simulink model "test4"  (R2015a)
settings: Solver=ode45  StartTime=0.0  StopTime=330000  RelTol=1e-3
InitFcn:
  | %% DSPBuilder Start
  | alt_dspbuilder_update_model(bdroot)
  | %% DSPBuilder End
libraries: allblocks_alteradspbuilder2 x840
(part 2 of 11)

== system test4/sift/Subsystem1/calculate_key_point/find_KeyPoint ==
  dataIn_10 : Inport
  dataIn_11 : Inport  Port=2
  dataIn_12 : Inport  Port=3
  dataIn_13 : Inport  Port=4
  dataIn_14 : Inport  Port=5
  dataIn_15 : Inport  Port=6
  dataIn_16 : Inport  Port=7
  dataIn_17 : Inport  Port=8
  dataIn_18 : Inport  Port=9
  dataIn_20 : Inport  Port=10
  dataIn_21 : Inport  Port=11
  dataIn_22 : Inport  Port=12
  dataIn_23 : Inport  Port=13
  dataIn_24 : Inport  Port=14
  dataIn_25 : Inport  Port=15
  dataIn_26 : Inport  Port=16
  dataIn_27 : Inport  Port=17
  dataIn_28 : Inport  Port=18
  dataIn_30 : Inport  Port=19
  dataIn_31 : Inport  Port=20
  dataIn_32 : Inport  Port=21
  dataIn_33 : Inport  Port=22
  dataIn_34 : Inport  Port=23
  dataIn_35 : Inport  Port=24
  dataIn_36 : Inport  Port=25
  dataIn_37 : Inport  Port=26
  dataIn_38 : Inport  Port=27
  Logical Bit Operator : allblocks_alteradspbuilder2/Logical Bit Operator  LogicalOperator=OR  user_inputs=2  pipeline_display=0
  find_Keymax : Subsystem
  find_min : Subsystem
  is_KeyPoint : Outport
  wires:
  [dataIn_32] -> find_Keymax/21(dataIn_32)
  [dataIn_33] -> find_Keymax/22(dataIn_33)
  [dataIn_36] -> find_Keymax/25(dataIn_36)
  [dataIn_37] -> find_Keymax/26(dataIn_37)
  [dataIn_34] -> find_Keymax/23(dataIn_34)
  [dataIn_35] -> find_Keymax/24(dataIn_35)
  [dataIn_30] -> find_Keymax/19(dataIn_30)
  [dataIn_31] -> find_Keymax/20(dataIn_31)
  [is_KeyPoint_Max] -> Logical Bit Operator/2
  [is_KeyPoint_Min] -> Logical Bit Operator/1
  find_Keymax/1(is_KeyPoint) -> [is_KeyPoint_Max]
  [dataIn_28] -> find_Keymax/18(dataIn_28)
  [dataIn_26] -> find_Keymax/16(dataIn_26)
  [dataIn_22] -> find_Keymax/12(dataIn_22)
  [dataIn_27] -> find_Keymax/17(dataIn_27)
  [dataIn_20] -> find_Keymax/10(dataIn_20)
  [dataIn_23] -> find_Keymax/13(dataIn_23)
  [dataIn_24] -> find_Keymax/14(dataIn_24)
  [dataIn_21] -> find_Keymax/11(dataIn_21)
  [dataIn_25] -> find_Keymax/15(dataIn_25)
  [dataIn_10] -> find_Keymax/1(dataIn_10)
  [dataIn_11] -> find_Keymax/2(dataIn_11)
  [dataIn_12] -> find_Keymax/3(dataIn_12)
  dataIn_23/1 -> [dataIn_23]
  dataIn_17/1 -> [dataIn_17]
  dataIn_22/1 -> [dataIn_22]
  dataIn_14/1 -> [dataIn_14]
  dataIn_16/1 -> [dataIn_16]
  dataIn_28/1 -> [dataIn_28]
  dataIn_20/1 -> [dataIn_20]
  dataIn_21/1 -> [dataIn_21]
  dataIn_26/1 -> [dataIn_26]
  dataIn_10/1 -> [dataIn_10]
  dataIn_30/1 -> [dataIn_30]
  dataIn_27/1 -> [dataIn_27]
  dataIn_25/1 -> [dataIn_25]
  dataIn_15/1 -> [dataIn_15]
  dataIn_18/1 -> [dataIn_18]
  dataIn_24/1 -> [dataIn_24]
  dataIn_32/1 -> [dataIn_32]
  dataIn_13/1 -> [dataIn_13]
  dataIn_31/1 -> [dataIn_31]
  [dataIn_14] -> find_Keymax/5(dataIn_14)
  dataIn_34/1 -> [dataIn_34]
  dataIn_11/1 -> [dataIn_11]
  [dataIn_17] -> find_Keymax/8(dataIn_17)
  dataIn_35/1 -> [dataIn_35]
  dataIn_33/1 -> [dataIn_33]
  dataIn_38/1 -> [dataIn_38]
  [dataIn_13] -> find_Keymax/4(dataIn_13)
  [dataIn_16] -> find_Keymax/7(dataIn_16)
  [dataIn_15] -> find_Keymax/6(dataIn_15)
  dataIn_12/1 -> [dataIn_12]
  [dataIn_18] -> find_Keymax/9(dataIn_18)
  dataIn_36/1 -> [dataIn_36]
  dataIn_37/1 -> [dataIn_37]
  [dataIn_38] -> find_Keymax/27(dataIn_38)
  find_min/1(is_KeyPoint) -> [is_KeyPoint_Min]
  [dataIn_11] -> find_min/2(dataIn_11)
  [dataIn_12] -> find_min/3(dataIn_12)
  [dataIn_13] -> find_min/4(dataIn_13)
  [dataIn_15] -> find_min/6(dataIn_15)
  [dataIn_16] -> find_min/7(dataIn_16)
  [dataIn_17] -> find_min/8(dataIn_17)
  [dataIn_18] -> find_min/9(dataIn_18)
  [dataIn_31] -> find_min/20(dataIn_31)
  [dataIn_14] -> find_min/5(dataIn_14)
  [is_KeyPoint] -> is_KeyPoint/1
  [dataIn_33] -> find_min/22(dataIn_33)
  [dataIn_32] -> find_min/21(dataIn_32)
  [dataIn_34] -> find_min/23(dataIn_34)
  [dataIn_35] -> find_min/24(dataIn_35)
  [dataIn_36] -> find_min/25(dataIn_36)
  [dataIn_21] -> find_min/11(dataIn_21)
  [dataIn_22] -> find_min/12(dataIn_22)
  [dataIn_23] -> find_min/13(dataIn_23)
  [dataIn_25] -> find_min/15(dataIn_25)
  [dataIn_24] -> find_min/14(dataIn_24)
  [dataIn_38] -> find_min/27(dataIn_38)
  [dataIn_20] -> find_min/10(dataIn_20)
  [dataIn_26] -> find_min/16(dataIn_26)
  [dataIn_30] -> find_min/19(dataIn_30)
  [dataIn_27] -> find_min/17(dataIn_27)
  [dataIn_37] -> find_min/26(dataIn_37)
  [dataIn_28] -> find_min/18(dataIn_28)
  [dataIn_10] -> find_min/1(dataIn_10)
  Logical Bit Operator/1 -> [is_KeyPoint]

== system test4/sift/Subsystem1/calculate_key_point/line_buff_3x3 ==
  dataIn : Inport
  clken : Inport  Port=2
  Delay : allblocks_alteradspbuilder2/Delay  pipeline=1  pipeline_display=1  ClockPhase=1  use_ena=on  use_sclr=off  allowFloatingPointOverride=on  logOutputs=off  logFile=C:\Users\ASUS\Desktop\sift_fpga_final\Octave_2\tb_test4\test4_sift_Subsystem1_calculate%5Fkey%5Fpoint_line%5Fbuff%5F3x3_Delay.fixedpointlog  use_init=off  reset_value=1
  Delay1 : allblocks_alteradspbuilder2/Delay  pipeline=1  pipeline_display=1  ClockPhase=1  use_ena=on  use_sclr=off  allowFloatingPointOverride=on  logOutputs=off  logFile=C:\Users\ASUS\Desktop\sift_fpga_final\Octave_2\tb_test4\test4_sift_Subsystem1_calculate%5Fkey%5Fpoint_line%5Fbuff%5F3x3_Delay1.fixedpointlog  use_init=off  reset_value=1
  Delay10 : allblocks_alteradspbuilder2/Delay  pipeline=1  pipeline_display=1  ClockPhase=1  use_ena=on  use_sclr=off  allowFloatingPointOverride=on  logOutputs=off  logFile=C:\Users\ASUS\Desktop\sift_fpga_final\Octave_2\tb_test4\test4_sift_Subsystem1_calculate%5Fkey%5Fpoint_line%5Fbuff%5F3x3_Delay10.fixedpointlog  use_init=off  reset_value=1
  Delay2 : allblocks_alteradspbuilder2/Delay  pipeline=1  pipeline_display=1  ClockPhase=1  use_ena=on  use_sclr=off  allowFloatingPointOverride=on  logOutputs=off  logFile=C:\Users\ASUS\Desktop\sift_fpga_final\Octave_2\tb_test4\test4_sift_Subsystem1_calculate%5Fkey%5Fpoint_line%5Fbuff%5F3x3_Delay2.fixedpointlog  use_init=off  reset_value=1
  Delay5 : allblocks_alteradspbuilder2/Delay  pipeline=1  pipeline_display=1  ClockPhase=1  use_ena=on  use_sclr=off  allowFloatingPointOverride=on  logOutputs=off  logFile=C:\Users\ASUS\Desktop\sift_fpga_final\Octave_2\tb_test4\test4_sift_Subsystem1_calculate%5Fkey%5Fpoint_line%5Fbuff%5F3x3_Delay5.fixedpointlog  use_init=off  reset_value=1
  Delay6 : allblocks_alteradspbuilder2/Delay  pipeline=1  pipeline_display=1  ClockPhase=1  use_ena=on  use_sclr=off  allowFloatingPointOverride=on  logOutputs=off  logFile=C:\Users\ASUS\Desktop\sift_fpga_final\Octave_2\tb_test4\test4_sift_Subsystem1_calculate%5Fkey%5Fpoint_line%5Fbuff%5F3x3_Delay6.fixedpointlog  use_init=off  reset_value=1
  Delay9 : allblocks_alteradspbuilder2/Delay  pipeline=1  pipeline_display=1  ClockPhase=1  use_ena=on  use_sclr=off  allowFloatingPointOverride=on  logOutputs=off  logFile=C:\Users\ASUS\Desktop\sift_fpga_final\Octave_2\tb_test4\test4_sift_Subsystem1_calculate%5Fkey%5Fpoint_line%5Fbuff%5F3x3_Delay9.fixedpointlog  use_init=off  reset_value=1
  Memory Delay : allblocks_alteradspbuilder2/Memory Delay  BusType=Signed Integer  bwl=9  bwr=16  pipeline=318  pipeline_display=318  ram_type=AUTO  use_ena=on  use_sclr=off  allowFloatingPointOverride=on  logOutputs=off  logFile=C:\Users\ASUS\Desktop\sift_fpga_final\Octave_2\tb_test4\test4_sift_Subsystem1_calculate%5Fkey%5Fpoint_line%5Fbuff%5F3x3_Memory+Delay.fixedpointlog
  Memory Delay1 : allblocks_alteradspbuilder2/Memory Delay  BusType=Signed Integer  bwl=9  bwr=16  pipeline=318  pipeline_display=318  ram_type=AUTO  use_ena=on  use_sclr=off  allowFloatingPointOverride=on  logOutputs=off  logFile=C:\Users\ASUS\Desktop\sift_fpga_final\Octave_2\tb_test4\test4_sift_Subsystem1_calculate%5Fkey%5Fpoint_line%5Fbuff%5F3x3_Memory+Delay1.fixedpointlog
  Out00 : Outport
  Out01 : Outport  Port=2
  Out02 : Outport  Port=3
  Out10 : Outport  Port=4
  Out11 : Outport  Port=5
  Out12 : Outport  Port=6
  Out20 : Outport  Port=7
  Out21 : Outport  Port=8
  Out22 : Outport  Port=9
  wires:
  Delay1/1 -> [data_01], Delay2/1
  Delay/1 -> [data_00], Delay1/1
  Delay9/1 -> [data_21], Delay10/1
  [clken] -> Delay10/2
  [clken] -> Memory Delay1/2
  Delay6/1 -> Memory Delay1/1, [data_12]
  Memory Delay1/1 -> [data_20], Delay9/1
  [clken] -> Delay9/2
  [data_02] -> Out02/1
  [clken] -> Delay1/2
  [clken] -> Delay/2
  [data_in] -> Delay/1
  [clken] -> Delay2/2
  Delay2/1 -> Memory Delay/1, [data_02]
  [data_22] -> Out22/1
  Delay10/1 -> [data_22]
  clken/1 -> [clken]
  [data_21] -> Out21/1
  [data_20] -> Out20/1
  [data_10] -> Out10/1
  Memory Delay/1 -> [data_10], Delay5/1
  [clken] -> Memory Delay/2
  [clken] -> Delay6/2
  Delay5/1 -> [data_11], Delay6/1
  [data_12] -> Out12/1
  [data_00] -> Out00/1
  [data_01] -> Out01/1
  [clken] -> Delay5/2
  [data_11] -> Out11/1
  dataIn/1 -> [data_in]

== system test4/sift/Subsystem1/calculate_key_point/line_buff_3x3(1) ==
  dataIn : Inport
  clken : Inport  Port=2
  Delay : allblocks_alteradspbuilder2/Delay  pipeline=1  pipeline_display=1  ClockPhase=1  use_ena=on  use_sclr=off  allowFloatingPointOverride=on  logOutputs=off  logFile=C:\Users\ASUS\Desktop\sift_fpga_final\Octave_2\tb_test4\test4_sift_Subsystem1_calculate%5Fkey%5Fpoint_line%5Fbuff%5F3x3%281%29_Delay.fixedpointlog  use_init=off  reset_value=1
  Delay1 : allblocks_alteradspbuilder2/Delay  pipeline=1  pipeline_display=1  ClockPhase=1  use_ena=on  use_sclr=off  allowFloatingPointOverride=on  logOutputs=off  logFile=C:\Users\ASUS\Desktop\sift_fpga_final\Octave_2\tb_test4\test4_sift_Subsystem1_calculate%5Fkey%5Fpoint_line%5Fbuff%5F3x3%281%29_Delay1.fixedpointlog  use_init=off  reset_value=1
  Delay10 : allblocks_alteradspbuilder2/Delay  pipeline=1  pipeline_display=1  ClockPhase=1  use_ena=on  use_sclr=off  allowFloatingPointOverride=on  logOutputs=off  logFile=C:\Users\ASUS\Desktop\sift_fpga_final\Octave_2\tb_test4\test4_sift_Subsystem1_calculate%5Fkey%5Fpoint_line%5Fbuff%5F3x3%281%29_Delay10.fixedpointlog  use_init=off  reset_value=1
  Delay2 : allblocks_alteradspbuilder2/Delay  pipeline=1  pipeline_display=1  ClockPhase=1  use_ena=on  use_sclr=off  allowFloatingPointOverride=on  logOutputs=off  logFile=C:\Users\ASUS\Desktop\sift_fpga_final\Octave_2\tb_test4\test4_sift_Subsystem1_calculate%5Fkey%5Fpoint_line%5Fbuff%5F3x3%281%29_Delay2.fixedpointlog  use_init=off  reset_value=1
  Delay5 : allblocks_alteradspbuilder2/Delay  pipeline=1  pipeline_display=1  ClockPhase=1  use_ena=on  use_sclr=off  allowFloatingPointOverride=on  logOutputs=off  logFile=C:\Users\ASUS\Desktop\sift_fpga_final\Octave_2\tb_test4\test4_sift_Subsystem1_calculate%5Fkey%5Fpoint_line%5Fbuff%5F3x3%281%29_Delay5.fixedpointlog  use_init=off  reset_value=1
  Delay6 : allblocks_alteradspbuilder2/Delay  pipeline=1  pipeline_display=1  ClockPhase=1  use_ena=on  use_sclr=off  allowFloatingPointOverride=on  logOutputs=off  logFile=C:\Users\ASUS\Desktop\sift_fpga_final\Octave_2\tb_test4\test4_sift_Subsystem1_calculate%5Fkey%5Fpoint_line%5Fbuff%5F3x3%281%29_Delay6.fixedpointlog  use_init=off  reset_value=1
  Delay9 : allblocks_alteradspbuilder2/Delay  pipeline=1  pipeline_display=1  ClockPhase=1  use_ena=on  use_sclr=off  allowFloatingPointOverride=on  logOutputs=off  logFile=C:\Users\ASUS\Desktop\sift_fpga_final\Octave_2\tb_test4\test4_sift_Subsystem1_calculate%5Fkey%5Fpoint_line%5Fbuff%5F3x3%281%29_Delay9.fixedpointlog  use_init=off  reset_value=1
  Memory Delay : allblocks_alteradspbuilder2/Memory Delay  BusType=Signed Integer  bwl=9  bwr=16  pipeline=318  pipeline_display=318  ram_type=AUTO  use_ena=on  use_sclr=off  allowFloatingPointOverride=on  logOutputs=off  logFile=C:\Users\ASUS\Desktop\sift_fpga_final\Octave_2\tb_test4\test4_sift_Subsystem1_calculate%5Fkey%5Fpoint_line%5Fbuff%5F3x3%281%29_Memory+Delay.fixedpointlog
  Memory Delay1 : allblocks_alteradspbuilder2/Memory Delay  BusType=Signed Integer  bwl=9  bwr=16  pipeline=318  pipeline_display=318  ram_type=AUTO  use_ena=on  use_sclr=off  allowFloatingPointOverride=on  logOutputs=off  logFile=C:\Users\ASUS\Desktop\sift_fpga_final\Octave_2\tb_test4\test4_sift_Subsystem1_calculate%5Fkey%5Fpoint_line%5Fbuff%5F3x3%281%29_Memory+Delay1.fixedpointlog
  Out00 : Outport
  Out01 : Outport  Port=2
  Out02 : Outport  Port=3
  Out10 : Outport  Port=4
  Out11 : Outport  Port=5
  Out12 : Outport  Port=6
  Out20 : Outport  Port=7
  Out21 : Outport  Port=8
  Out22 : Outport  Port=9
  wires:
  Delay1/1 -> [data_01], Delay2/1
  Delay/1 -> [data_00], Delay1/1
  Delay9/1 -> [data_21], Delay10/1
  [clken] -> Delay10/2
  [clken] -> Memory Delay1/2
  Delay6/1 -> Memory Delay1/1, [data_12]
  Memory Delay1/1 -> [data_20], Delay9/1
  [clken] -> Delay9/2
  [data_02] -> Out02/1
  [clken] -> Delay1/2
  [clken] -> Delay/2
  [data_in] -> Delay/1
  [clken] -> Delay2/2
  Delay2/1 -> Memory Delay/1, [data_02]
  [data_22] -> Out22/1
  Delay10/1 -> [data_22]
  clken/1 -> [clken]
  [data_21] -> Out21/1
  [data_20] -> Out20/1
  [data_10] -> Out10/1
  Memory Delay/1 -> [data_10], Delay5/1
  [clken] -> Memory Delay/2
  [clken] -> Delay6/2
  Delay5/1 -> [data_11], Delay6/1
  [data_12] -> Out12/1
  [data_00] -> Out00/1
  [data_01] -> Out01/1
  [clken] -> Delay5/2
  [data_11] -> Out11/1
  dataIn/1 -> [data_in]

== system test4/sift/Subsystem1/calculate_key_point/line_buff_3x3(2) ==
  dataIn : Inport
  clken : Inport  Port=2
  Delay : allblocks_alteradspbuilder2/Delay  pipeline=1  pipeline_display=1  ClockPhase=1  use_ena=on  use_sclr=off  allowFloatingPointOverride=on  logOutputs=off  logFile=C:\Users\ASUS\Desktop\sift_fpga_final\Octave_2\tb_test4\test4_sift_Subsystem1_calculate%5Fkey%5Fpoint_line%5Fbuff%5F3x3%282%29_Delay.fixedpointlog  use_init=off  reset_value=1
  Delay1 : allblocks_alteradspbuilder2/Delay  pipeline=1  pipeline_display=1  ClockPhase=1  use_ena=on  use_sclr=off  allowFloatingPointOverride=on  logOutputs=off  logFile=C:\Users\ASUS\Desktop\sift_fpga_final\Octave_2\tb_test4\test4_sift_Subsystem1_calculate%5Fkey%5Fpoint_line%5Fbuff%5F3x3%282%29_Delay1.fixedpointlog  use_init=off  reset_value=1
  Delay10 : allblocks_alteradspbuilder2/Delay  pipeline=1  pipeline_display=1  ClockPhase=1  use_ena=on  use_sclr=off  allowFloatingPointOverride=on  logOutputs=off  logFile=C:\Users\ASUS\Desktop\sift_fpga_final\Octave_2\tb_test4\test4_sift_Subsystem1_calculate%5Fkey%5Fpoint_line%5Fbuff%5F3x3%282%29_Delay10.fixedpointlog  use_init=off  reset_value=1
  Delay2 : allblocks_alteradspbuilder2/Delay  pipeline=1  pipeline_display=1  ClockPhase=1  use_ena=on  use_sclr=off  allowFloatingPointOverride=on  logOutputs=off  logFile=C:\Users\ASUS\Desktop\sift_fpga_final\Octave_2\tb_test4\test4_sift_Subsystem1_calculate%5Fkey%5Fpoint_line%5Fbuff%5F3x3%282%29_Delay2.fixedpointlog  use_init=off  reset_value=1
  Delay5 : allblocks_alteradspbuilder2/Delay  pipeline=1  pipeline_display=1  ClockPhase=1  use_ena=on  use_sclr=off  allowFloatingPointOverride=on  logOutputs=off  logFile=C:\Users\ASUS\Desktop\sift_fpga_final\Octave_2\tb_test4\test4_sift_Subsystem1_calculate%5Fkey%5Fpoint_line%5Fbuff%5F3x3%282%29_Delay5.fixedpointlog  use_init=off  reset_value=1
  Delay6 : allblocks_alteradspbuilder2/Delay  pipeline=1  pipeline_display=1  ClockPhase=1  use_ena=on  use_sclr=off  allowFloatingPointOverride=on  logOutputs=off  logFile=C:\Users\ASUS\Desktop\sift_fpga_final\Octave_2\tb_test4\test4_sift_Subsystem1_calculate%5Fkey%5Fpoint_line%5Fbuff%5F3x3%282%29_Delay6.fixedpointlog  use_init=off  reset_value=1
  Delay9 : allblocks_alteradspbuilder2/Delay  pipeline=1  pipeline_display=1  ClockPhase=1  use_ena=on  use_sclr=off  allowFloatingPointOverride=on  logOutputs=off  logFile=C:\Users\ASUS\Desktop\sift_fpga_final\Octave_2\tb_test4\test4_sift_Subsystem1_calculate%5Fkey%5Fpoint_line%5Fbuff%5F3x3%282%29_Delay9.fixedpointlog  use_init=off  reset_value=1
  Memory Delay : allblocks_alteradspbuilder2/Memory Delay  BusType=Signed Integer  bwl=9  bwr=16  pipeline=318  pipeline_display=318  ram_type=AUTO  use_ena=on  use_sclr=off  allowFloatingPointOverride=on  logOutputs=off  logFile=C:\Users\ASUS\Desktop\sift_fpga_final\Octave_2\tb_test4\test4_sift_Subsystem1_calculate%5Fkey%5Fpoint_line%5Fbuff%5F3x3%282%29_Memory+Delay.fixedpointlog
  Memory Delay1 : allblocks_alteradspbuilder2/Memory Delay  BusType=Signed Integer  bwl=9  bwr=16  pipeline=318  pipeline_display=318  ram_type=AUTO  use_ena=on  use_sclr=off  allowFloatingPointOverride=on  logOutputs=off  logFile=C:\Users\ASUS\Desktop\sift_fpga_final\Octave_2\tb_test4\test4_sift_Subsystem1_calculate%5Fkey%5Fpoint_line%5Fbuff%5F3x3%282%29_Memory+Delay1.fixedpointlog
  Out00 : Outport
  Out01 : Outport  Port=2
  Out02 : Outport  Port=3
  Out10 : Outport  Port=4
  Out11 : Outport  Port=5
  Out12 : Outport  Port=6
  Out20 : Outport  Port=7
  Out21 : Outport  Port=8
  Out22 : Outport  Port=9
  wires:
  Delay1/1 -> [data_01], Delay2/1
  Delay/1 -> [data_00], Delay1/1
  Delay9/1 -> [data_21], Delay10/1
  [clken] -> Delay10/2
  [clken] -> Memory Delay1/2
  Delay6/1 -> Memory Delay1/1, [data_12]
  Memory Delay1/1 -> [data_20], Delay9/1
  [clken] -> Delay9/2
  [data_02] -> Out02/1
  [clken] -> Delay1/2
  [clken] -> Delay/2
  [data_in] -> Delay/1
  [clken] -> Delay2/2
  Delay2/1 -> Memory Delay/1, [data_02]
  [data_22] -> Out22/1
  Delay10/1 -> [data_22]
  clken/1 -> [clken]
  [data_21] -> Out21/1
  [data_20] -> Out20/1
  [data_10] -> Out10/1
  Memory Delay/1 -> [data_10], Delay5/1
  [clken] -> Memory Delay/2
  [clken] -> Delay6/2
  Delay5/1 -> [data_11], Delay6/1
  [data_12] -> Out12/1
  [data_00] -> Out00/1
  [data_01] -> Out01/1
  [clken] -> Delay5/2
  [data_11] -> Out11/1
  dataIn/1 -> [data_in]

== system test4/sift/Subsystem1/scale_space/Gaussian_scale1 ==
  pixel_in : Inport
  valid_in : Inport  Port=2
  Mul : Subsystem
  Round : allblocks_alteradspbuilder2/Round  BusType=Signed Fractional  bwl=9  bwr=16  bitsToRemove=0  roundMode=TRUNCATE_LOW  userRoundMode=Truncate  pipeline=off  pipeline_display=0  use_ena=off  use_aclr=off
  line_buff : Subsystem
  pixel_out : Outport
  wires:
  line_buff/20(Out34) -> Mul/20(In34)
  line_buff/7(Out11) -> Mul/7(In11)
  line_buff/22(Out41) -> Mul/22(In41)
  line_buff/21(Out40) -> Mul/21(In40)
  line_buff/23(Out42) -> Mul/23(In42)
  line_buff/24(Out43) -> Mul/24(In43)
  line_buff/6(Out10) -> Mul/6(In10)
  line_buff/19(Out33) -> Mul/19(In33)
  line_buff/25(Out44) -> Mul/25(In44)
  line_buff/11(Out20) -> Mul/11(In20)
  line_buff/1(Out00) -> Mul/1(In00)
  line_buff/5(Out04) -> Mul/5(In04)
  pixel_in/1 -> line_buff/1(dataIn)
  line_buff/13(Out22) -> Mul/13(In22)
  line_buff/16(Out30) -> Mul/16(In30)
  line_buff/18(Out32) -> Mul/18(In32)
  Mul/1(pixel) -> Round/1
  line_buff/10(Out14) -> Mul/10(In14)
  valid_in/1 -> Mul/26(clken), line_buff/2(clken)
  line_buff/12(Out21) -> Mul/12(In21)
  line_buff/14(Out23) -> Mul/14(In23)
  line_buff/2(Out01) -> Mul/2(In01)
  line_buff/4(Out03) -> Mul/4(In03)
  line_buff/9(Out13) -> Mul/9(In13)
  line_buff/15(Out24) -> Mul/15(In24)
  line_buff/17(Out31) -> Mul/17(In31)
  line_buff/3(Out02) -> Mul/3(In02)
  line_buff/8(Out12) -> Mul/8(In12)
  Round/1 -> pixel_out/1

== system test4/sift/Subsystem1/scale_space/Gaussian_scale2 ==
  pixel_in : Inport
  valid_in : Inport  Port=2
  Mul : Subsystem
  Round : allblocks_alteradspbuilder2/Round  BusType=Signed Fractional  bwl=9  bwr=16  bitsToRemove=0  roundMode=TRUNCATE_LOW  userRoundMode=Truncate  pipeline=off  pipeline_display=0  use_ena=off  use_aclr=off
  line_buff : Subsystem
  pixel_out : Outport
  wires:
  line_buff/20(Out34) -> Mul/20(In34)
  line_buff/7(Out11) -> Mul/7(In11)
  line_buff/22(Out41) -> Mul/22(In41)
  line_buff/21(Out40) -> Mul/21(In40)
  line_buff/23(Out42) -> Mul/23(In42)
  line_buff/24(Out43) -> Mul/24(In43)
  line_buff/6(Out10) -> Mul/6(In10)
  line_buff/19(Out33) -> Mul/19(In33)
  line_buff/25(Out44) -> Mul/25(In44)
  line_buff/11(Out20) -> Mul/11(In20)
  line_buff/1(Out00) -> Mul/1(In00)
  line_buff/5(Out04) -> Mul/5(In04)
  pixel_in/1 -> line_buff/1(dataIn)
  line_buff/13(Out22) -> Mul/13(In22)
  line_buff/16(Out30) -> Mul/16(In30)
  line_buff/18(Out32) -> Mul/18(In32)
  Mul/1(pixel) -> Round/1
  line_buff/10(Out14) -> Mul/10(In14)
  valid_in/1 -> Mul/26(clken), line_buff/2(clken)
  line_buff/12(Out21) -> Mul/12(In21)
  line_buff/14(Out23) -> Mul/14(In23)
  line_buff/2(Out01) -> Mul/2(In01)
  line_buff/4(Out03) -> Mul/4(In03)
  line_buff/9(Out13) -> Mul/9(In13)
  line_buff/15(Out24) -> Mul/15(In24)
  line_buff/17(Out31) -> Mul/17(In31)
  line_buff/3(Out02) -> Mul/3(In02)
  line_buff/8(Out12) -> Mul/8(In12)
  Round/1 -> pixel_out/1

== system test4/sift/Subsystem1/scale_space/Gaussian_scale3 ==
  pixel_in : Inport
  valid_in : Inport  Port=2
  Mul : Subsystem
  Round : allblocks_alteradspbuilder2/Round  BusType=Signed Fractional  bwl=9  bwr=16  bitsToRemove=0  roundMode=TRUNCATE_LOW  userRoundMode=Truncate  pipeline=off  pipeline_display=0  use_ena=off  use_aclr=off
  line_buff : Subsystem
  pixel_out : Outport
  wires:
  line_buff/20(Out34) -> Mul/20(In34)
  line_buff/7(Out11) -> Mul/7(In11)
  line_buff/22(Out41) -> Mul/22(In41)
  line_buff/21(Out40) -> Mul/21(In40)
  line_buff/23(Out42) -> Mul/23(In42)
  line_buff/24(Out43) -> Mul/24(In43)
  line_buff/6(Out10) -> Mul/6(In10)
  line_buff/19(Out33) -> Mul/19(In33)
  line_buff/25(Out44) -> Mul/25(In44)
  line_buff/11(Out20) -> Mul/11(In20)
  line_buff/1(Out00) -> Mul/1(In00)
  line_buff/5(Out04) -> Mul/5(In04)
  pixel_in/1 -> line_buff/1(dataIn)
  line_buff/13(Out22) -> Mul/13(In22)
  line_buff/16(Out30) -> Mul/16(In30)
  line_buff/18(Out32) -> Mul/18(In32)
  Mul/1(pixel) -> Round/1
  line_buff/10(Out14) -> Mul/10(In14)
  valid_in/1 -> Mul/26(clken), line_buff/2(clken)
  line_buff/12(Out21) -> Mul/12(In21)
  line_buff/14(Out23) -> Mul/14(In23)
  line_buff/2(Out01) -> Mul/2(In01)
  line_buff/4(Out03) -> Mul/4(In03)
  line_buff/9(Out13) -> Mul/9(In13)
  line_buff/15(Out24) -> Mul/15(In24)
  line_buff/17(Out31) -> Mul/17(In31)
  line_buff/3(Out02) -> Mul/3(In02)
  line_buff/8(Out12) -> Mul/8(In12)
  Round/1 -> pixel_out/1

== system test4/sift/Subsystem1/scale_space/Gaussian_scale4 ==
  pixel_in : Inport
  valid_in : Inport  Port=2
  Mul : Subsystem
  Round : allblocks_alteradspbuilder2/Round  BusType=Signed Fractional  bwl=9  bwr=16  bitsToRemove=0  roundMode=TRUNCATE_LOW  userRoundMode=Truncate  pipeline=off  pipeline_display=0  use_ena=off  use_aclr=off
  line_buff : Subsystem
  pixel_out : Outport
  wires:
  line_buff/20(Out34) -> Mul/20(In34)
  line_buff/7(Out11) -> Mul/7(In11)
  line_buff/22(Out41) -> Mul/22(In41)
  line_buff/21(Out40) -> Mul/21(In40)
  line_buff/23(Out42) -> Mul/23(In42)
  line_buff/24(Out43) -> Mul/24(In43)
  line_buff/6(Out10) -> Mul/6(In10)
  line_buff/19(Out33) -> Mul/19(In33)
  line_buff/25(Out44) -> Mul/25(In44)
  line_buff/11(Out20) -> Mul/11(In20)
  line_buff/1(Out00) -> Mul/1(In00)
  line_buff/5(Out04) -> Mul/5(In04)
  pixel_in/1 -> line_buff/1(dataIn)
  line_buff/13(Out22) -> Mul/13(In22)
  line_buff/16(Out30) -> Mul/16(In30)
  line_buff/18(Out32) -> Mul/18(In32)
  Mul/1(pixel) -> Round/1
  line_buff/10(Out14) -> Mul/10(In14)
  valid_in/1 -> Mul/26(clken), line_buff/2(clken)
  line_buff/12(Out21) -> Mul/12(In21)
  line_buff/14(Out23) -> Mul/14(In23)
  line_buff/2(Out01) -> Mul/2(In01)
  line_buff/4(Out03) -> Mul/4(In03)
  line_buff/9(Out13) -> Mul/9(In13)
  line_buff/15(Out24) -> Mul/15(In24)
  line_buff/17(Out31) -> Mul/17(In31)
  line_buff/3(Out02) -> Mul/3(In02)
  line_buff/8(Out12) -> Mul/8(In12)
  Round/1 -> pixel_out/1

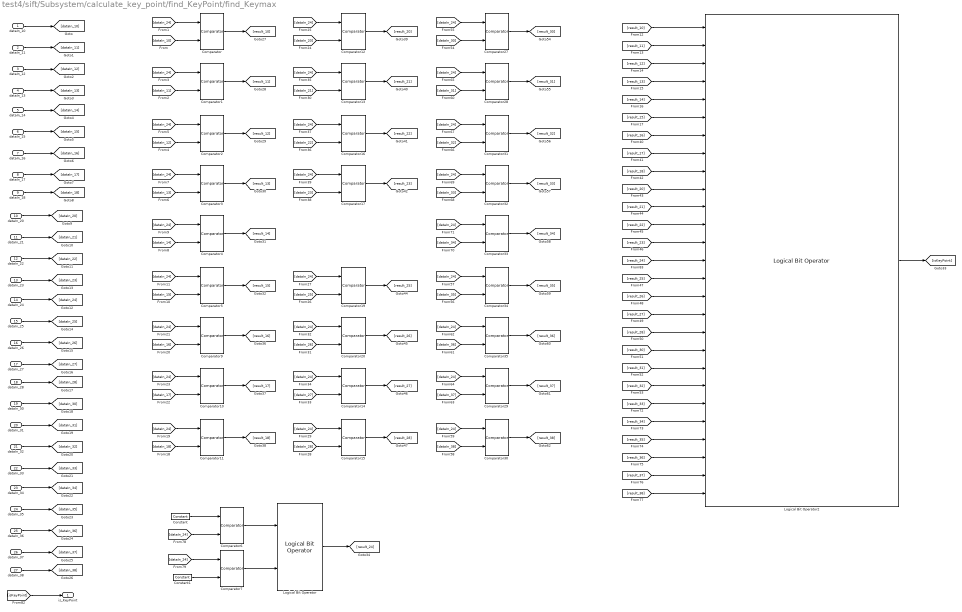
== system test4/sift/Subsystem/calculate_key_point/find_KeyPoint/find_Keymax ==
  dataIn_10 : Inport
  dataIn_11 : Inport  Port=2
  dataIn_12 : Inport  Port=3
  dataIn_13 : Inport  Port=4
  dataIn_14 : Inport  Port=5
  dataIn_15 : Inport  Port=6
  dataIn_16 : Inport  Port=7
  dataIn_17 : Inport  Port=8
  dataIn_18 : Inport  Port=9
  dataIn_20 : Inport  Port=10
  dataIn_21 : Inport  Port=11
  dataIn_22 : Inport  Port=12
  dataIn_23 : Inport  Port=13
  dataIn_24 : Inport  Port=14
  dataIn_25 : Inport  Port=15
  dataIn_26 : Inport  Port=16
  dataIn_27 : Inport  Port=17
  dataIn_28 : Inport  Port=18
  dataIn_30 : Inport  Port=19
  dataIn_31 : Inport  Port=20
  dataIn_32 : Inport  Port=21
  dataIn_33 : Inport  Port=22
  dataIn_34 : Inport  Port=23
  dataIn_35 : Inport  Port=24
  dataIn_36 : Inport  Port=25
  dataIn_37 : Inport  Port=26
  dataIn_38 : Inport  Port=27
  Comparator : allblocks_alteradspbuilder2/Comparator  direction=a > b  pipeline_display=0  allowFloatingPointOverride=on  logOutputs=off  logFile=C:\Users\ASUS\Desktop\sift_fpga_final\Octave_2\tb_test4\test4_sift_Subsystem_calculate%5Fkey%5Fpoint_find%5FKeyPoint_find%5FKeymax_Comparator.fixedpointlog
  Comparator1 : allblocks_alteradspbuilder2/Comparator  direction=a > b  pipeline_display=0  allowFloatingPointOverride=on  logOutputs=off  logFile=C:\Users\ASUS\Desktop\sift_fpga_final\Octave_2\tb_test4\test4_sift_Subsystem_calculate%5Fkey%5Fpoint_find%5FKeyPoint_find%5FKeymax_Comparator1.fixedpointlog
  Comparator10 : allblocks_alteradspbuilder2/Comparator  direction=a > b  pipeline_display=0  allowFloatingPointOverride=on  logOutputs=off  logFile=C:\Users\ASUS\Desktop\sift_fpga_final\Octave_2\tb_test4\test4_sift_Subsystem_calculate%5Fkey%5Fpoint_find%5FKeyPoint_find%5FKeymax_Comparator10.fixedpointlog
  Comparator11 : allblocks_alteradspbuilder2/Comparator  direction=a > b  pipeline_display=0  allowFloatingPointOverride=on  logOutputs=off  logFile=C:\Users\ASUS\Desktop\sift_fpga_final\Octave_2\tb_test4\test4_sift_Subsystem_calculate%5Fkey%5Fpoint_find%5FKeyPoint_find%5FKeymax_Comparator11.fixedpointlog
  Comparator12 : allblocks_alteradspbuilder2/Comparator  direction=a > b  pipeline_display=0  allowFloatingPointOverride=on  logOutputs=off  logFile=C:\Users\ASUS\Desktop\sift_fpga_final\Octave_2\tb_test4\test4_sift_Subsystem_calculate%5Fkey%5Fpoint_find%5FKeyPoint_find%5FKeymax_Comparator12.fixedpointlog
  Comparator13 : allblocks_alteradspbuilder2/Comparator  direction=a > b  pipeline_display=0  allowFloatingPointOverride=on  logOutputs=off  logFile=C:\Users\ASUS\Desktop\sift_fpga_final\Octave_2\tb_test4\test4_sift_Subsystem_calculate%5Fkey%5Fpoint_find%5FKeyPoint_find%5FKeymax_Comparator13.fixedpointlog
  Comparator14 : allblocks_alteradspbuilder2/Comparator  direction=a > b  pipeline_display=0  allowFloatingPointOverride=on  logOutputs=off  logFile=C:\Users\ASUS\Desktop\sift_fpga_final\Octave_2\tb_test4\test4_sift_Subsystem_calculate%5Fkey%5Fpoint_find%5FKeyPoint_find%5FKeymax_Comparator14.fixedpointlog
  Comparator15 : allblocks_alteradspbuilder2/Comparator  direction=a > b  pipeline_display=0  allowFloatingPointOverride=on  logOutputs=off  logFile=C:\Users\ASUS\Desktop\sift_fpga_final\Octave_2\tb_test4\test4_sift_Subsystem_calculate%5Fkey%5Fpoint_find%5FKeyPoint_find%5FKeymax_Comparator15.fixedpointlog
  Comparator16 : allblocks_alteradspbuilder2/Comparator  direction=a > b  pipeline_display=0  allowFloatingPointOverride=on  logOutputs=off  logFile=C:\Users\ASUS\Desktop\sift_fpga_final\Octave_2\tb_test4\test4_sift_Subsystem_calculate%5Fkey%5Fpoint_find%5FKeyPoint_find%5FKeymax_Comparator16.fixedpointlog
  Comparator17 : allblocks_alteradspbuilder2/Comparator  direction=a > b  pipeline_display=0  allowFloatingPointOverride=on  logOutputs=off  logFile=C:\Users\ASUS\Desktop\sift_fpga_final\Octave_2\tb_test4\test4_sift_Subsystem_calculate%5Fkey%5Fpoint_find%5FKeyPoint_find%5FKeymax_Comparator17.fixedpointlog
  Comparator19 : allblocks_alteradspbuilder2/Comparator  direction=a > b  pipeline_display=0  allowFloatingPointOverride=on  logOutputs=off  logFile=C:\Users\ASUS\Desktop\sift_fpga_final\Octave_2\tb_test4\test4_sift_Subsystem_calculate%5Fkey%5Fpoint_find%5FKeyPoint_find%5FKeymax_Comparator19.fixedpointlog
  Comparator2 : allblocks_alteradspbuilder2/Comparator  direction=a > b  pipeline_display=0  allowFloatingPointOverride=on  logOutputs=off  logFile=C:\Users\ASUS\Desktop\sift_fpga_final\Octave_2\tb_test4\test4_sift_Subsystem_calculate%5Fkey%5Fpoint_find%5FKeyPoint_find%5FKeymax_Comparator2.fixedpointlog
  Comparator20 : allblocks_alteradspbuilder2/Comparator  direction=a > b  pipeline_display=0  allowFloatingPointOverride=on  logOutputs=off  logFile=C:\Users\ASUS\Desktop\sift_fpga_final\Octave_2\tb_test4\test4_sift_Subsystem_calculate%5Fkey%5Fpoint_find%5FKeyPoint_find%5FKeymax_Comparator20.fixedpointlog
  Comparator27 : allblocks_alteradspbuilder2/Comparator  direction=a > b  pipeline_display=0  allowFloatingPointOverride=on  logOutputs=off  logFile=C:\Users\ASUS\Desktop\sift_fpga_final\Octave_2\tb_test4\test4_sift_Subsystem_calculate%5Fkey%5Fpoint_find%5FKeyPoint_find%5FKeymax_Comparator27.fixedpointlog
  Comparator28 : allblocks_alteradspbuilder2/Comparator  direction=a > b  pipeline_display=0  allowFloatingPointOverride=on  logOutputs=off  logFile=C:\Users\ASUS\Desktop\sift_fpga_final\Octave_2\tb_test4\test4_sift_Subsystem_calculate%5Fkey%5Fpoint_find%5FKeyPoint_find%5FKeymax_Comparator28.fixedpointlog
  Comparator29 : allblocks_alteradspbuilder2/Comparator  direction=a > b  pipeline_display=0  allowFloatingPointOverride=on  logOutputs=off  logFile=C:\Users\ASUS\Desktop\sift_fpga_final\Octave_2\tb_test4\test4_sift_Subsystem_calculate%5Fkey%5Fpoint_find%5FKeyPoint_find%5FKeymax_Comparator29.fixedpointlog
  Comparator3 : allblocks_alteradspbuilder2/Comparator  direction=a > b  pipeline_display=0  allowFloatingPointOverride=on  logOutputs=off  logFile=C:\Users\ASUS\Desktop\sift_fpga_final\Octave_2\tb_test4\test4_sift_Subsystem_calculate%5Fkey%5Fpoint_find%5FKeyPoint_find%5FKeymax_Comparator3.fixedpointlog
  Comparator30 : allblocks_alteradspbuilder2/Comparator  direction=a > b  pipeline_display=0  allowFloatingPointOverride=on  logOutputs=off  logFile=C:\Users\ASUS\Desktop\sift_fpga_final\Octave_2\tb_test4\test4_sift_Subsystem_calculate%5Fkey%5Fpoint_find%5FKeyPoint_find%5FKeymax_Comparator30.fixedpointlog
  Comparator31 : allblocks_alteradspbuilder2/Comparator  direction=a > b  pipeline_display=0  allowFloatingPointOverride=on  logOutputs=off  logFile=C:\Users\ASUS\Desktop\sift_fpga_final\Octave_2\tb_test4\test4_sift_Subsystem_calculate%5Fkey%5Fpoint_find%5FKeyPoint_find%5FKeymax_Comparator31.fixedpointlog
  Comparator32 : allblocks_alteradspbuilder2/Comparator  direction=a > b  pipeline_display=0  allowFloatingPointOverride=on  logOutputs=off  logFile=C:\Users\ASUS\Desktop\sift_fpga_final\Octave_2\tb_test4\test4_sift_Subsystem_calculate%5Fkey%5Fpoint_find%5FKeyPoint_find%5FKeymax_Comparator32.fixedpointlog
  Comparator33 : allblocks_alteradspbuilder2/Comparator  direction=a > b  pipeline_display=0  allowFloatingPointOverride=on  logOutputs=off  logFile=C:\Users\ASUS\Desktop\sift_fpga_final\Octave_2\tb_test4\test4_sift_Subsystem_calculate%5Fkey%5Fpoint_find%5FKeyPoint_find%5FKeymax_Comparator33.fixedpointlog
  Comparator34 : allblocks_alteradspbuilder2/Comparator  direction=a > b  pipeline_display=0  allowFloatingPointOverride=on  logOutputs=off  logFile=C:\Users\ASUS\Desktop\sift_fpga_final\Octave_2\tb_test4\test4_sift_Subsystem_calculate%5Fkey%5Fpoint_find%5FKeyPoint_find%5FKeymax_Comparator34.fixedpointlog
  Comparator35 : allblocks_alteradspbuilder2/Comparator  direction=a > b  pipeline_display=0  allowFloatingPointOverride=on  logOutputs=off  logFile=C:\Users\ASUS\Desktop\sift_fpga_final\Octave_2\tb_test4\test4_sift_Subsystem_calculate%5Fkey%5Fpoint_find%5FKeyPoint_find%5FKeymax_Comparator35.fixedpointlog
  Comparator4 : allblocks_alteradspbuilder2/Comparator  direction=a > b  pipeline_display=0  allowFloatingPointOverride=on  logOutputs=off  logFile=C:\Users\ASUS\Desktop\sift_fpga_final\Octave_2\tb_test4\test4_sift_Subsystem_calculate%5Fkey%5Fpoint_find%5FKeyPoint_find%5FKeymax_Comparator4.fixedpointlog
  Comparator5 : allblocks_alteradspbuilder2/Comparator  direction=a > b  pipeline_display=0  allowFloatingPointOverride=on  logOutputs=off  logFile=C:\Users\ASUS\Desktop\sift_fpga_final\Octave_2\tb_test4\test4_sift_Subsystem_calculate%5Fkey%5Fpoint_find%5FKeyPoint_find%5FKeymax_Comparator5.fixedpointlog
  Comparator6 : allblocks_alteradspbuilder2/Comparator  direction=a < b  pipeline_display=0  allowFloatingPointOverride=on  logOutputs=off  logFile=C:\Users\ASUS\Desktop\sift_fpga_final\Octave_2\tb_test4\test4_sift_Subsystem_calculate%5Fkey%5Fpoint_find%5FKeyPoint_find%5FKeymax_Comparator6.fixedpointlog
  Comparator7 : allblocks_alteradspbuilder2/Comparator  direction=a < b  pipeline_display=0  allowFloatingPointOverride=on  logOutputs=off  logFile=C:\Users\ASUS\Desktop\sift_fpga_final\Octave_2\tb_test4\test4_sift_Subsystem_calculate%5Fkey%5Fpoint_find%5FKeyPoint_find%5FKeymax_Comparator7.fixedpointlog
  Comparator9 : allblocks_alteradspbuilder2/Comparator  direction=a > b  pipeline_display=0  allowFloatingPointOverride=on  logOutputs=off  logFile=C:\Users\ASUS\Desktop\sift_fpga_final\Octave_2\tb_test4\test4_sift_Subsystem_calculate%5Fkey%5Fpoint_find%5FKeyPoint_find%5FKeymax_Comparator9.fixedpointlog
  Constant : allblocks_alteradspbuilder2/Constant  mask_cst=0.8*0.015  BusType=Signed Fractional  bwl=9  bwr=16  roundMode=Truncate  satMode=Wrap  SpecifyClock=off  allowFloatingPointOverride=on  logOutputs=off  logFile=C:\Users\ASUS\Desktop\sift_fpga_final\Octave_2\tb_test4\test4_sift_Subsystem_calculate%5Fkey%5Fpoint_find%5FKeyPoint_find%5FKeymax_Constant.fixedpointlog
  Constant1 : allblocks_alteradspbuilder2/Constant  mask_cst=-0.8*0.015  BusType=Signed Fractional  bwl=9  bwr=16  roundMode=Truncate  satMode=Wrap  SpecifyClock=off  allowFloatingPointOverride=on  logOutputs=off  logFile=C:\Users\ASUS\Desktop\sift_fpga_final\Octave_2\tb_test4\test4_sift_Subsystem_calculate%5Fkey%5Fpoint_find%5FKeyPoint_find%5FKeymax_Constant1.fixedpointlog
  Logical Bit Operator : allblocks_alteradspbuilder2/Logical Bit Operator  LogicalOperator=OR  user_inputs=2  pipeline_display=0
  Logical Bit Operator2 : allblocks_alteradspbuilder2/Logical Bit Operator  LogicalOperator=AND  user_inputs=27  pipeline_display=0
  is_KeyPoint : Outport
  wires:
  dataIn_18/1 -> [dataIn_18]
  dataIn_10/1 -> [dataIn_10]
  [result_10] -> Logical Bit Operator2/1
  [dataIn_24] -> Comparator/1
  Comparator1/1 -> [result_11]
  [dataIn_10] -> Comparator/2
  [dataIn_24] -> Comparator1/1
  [dataIn_11] -> Comparator1/2
  [result_20] -> Logical Bit Operator2/10
  [result_11] -> Logical Bit Operator2/2
  [result_22] -> Logical Bit Operator2/12
  [result_23] -> Logical Bit Operator2/13
  Comparator7/1 -> Logical Bit Operator/2
  [dataIn_24] -> Comparator2/1
  [dataIn_24] -> Comparator6/2
  Comparator2/1 -> [result_12]
  [dataIn_12] -> Comparator2/2
  [result_21] -> Logical Bit Operator2/11
  [dataIn_24] -> Comparator9/1
  Comparator9/1 -> [result_16]
  [dataIn_24] -> Comparator10/1
  [dataIn_16] -> Comparator9/2
  Comparator10/1 -> [result_17]
  [dataIn_17] -> Comparator10/2
  [dataIn_24] -> Comparator11/1
  Comparator11/1 -> [result_18]
  [dataIn_18] -> Comparator11/2
  dataIn_14/1 -> [dataIn_14]
  dataIn_15/1 -> [dataIn_15]
  dataIn_17/1 -> [dataIn_17]
  dataIn_16/1 -> [dataIn_16]
  dataIn_24/1 -> [dataIn_24]
  dataIn_27/1 -> [dataIn_27]
  dataIn_28/1 -> [dataIn_28]
  dataIn_25/1 -> [dataIn_25]
  dataIn_22/1 -> [dataIn_22]
  dataIn_20/1 -> [dataIn_20]
  dataIn_21/1 -> [dataIn_21]
  dataIn_23/1 -> [dataIn_23]
  dataIn_26/1 -> [dataIn_26]
  dataIn_30/1 -> [dataIn_30]
  dataIn_31/1 -> [dataIn_31]
  dataIn_32/1 -> [dataIn_32]
  dataIn_33/1 -> [dataIn_33]
  dataIn_37/1 -> [dataIn_37]
  dataIn_35/1 -> [dataIn_35]
  dataIn_34/1 -> [dataIn_34]
  dataIn_36/1 -> [dataIn_36]
  dataIn_38/1 -> [dataIn_38]
  dataIn_11/1 -> [dataIn_11]
  [dataIn_24] -> Comparator7/1
  [dataIn_13] -> Comparator3/2
  Comparator3/1 -> [result_13]
  [dataIn_24] -> Comparator4/1
  [dataIn_24] -> Comparator3/1
  [dataIn_24] -> Comparator5/1
  Comparator5/1 -> [result_15]
  [dataIn_14] -> Comparator4/2
  [dataIn_15] -> Comparator5/2
  Comparator4/1 -> [result_14]
  [dataIn_24] -> Comparator27/1
  [dataIn_24] -> Comparator28/1
  [dataIn_24] -> Comparator31/1
  [dataIn_32] -> Comparator31/2
  [dataIn_24] -> Comparator32/1
  [dataIn_33] -> Comparator32/2
  [dataIn_24] -> Comparator33/1
  Comparator32/1 -> [result_33]
  Comparator27/1 -> [result_30]
  Comparator28/1 -> [result_31]
  Comparator31/1 -> [result_32]
  [dataIn_30] -> Comparator27/2
  [dataIn_31] -> Comparator28/2
  [dataIn_35] -> Comparator34/2
  Comparator35/1 -> [result_36]
  Comparator34/1 -> [result_35]
  [dataIn_34] -> Comparator33/2
  [dataIn_24] -> Comparator35/1
  Comparator29/1 -> [result_37]
  [dataIn_24] -> Comparator30/1
  [dataIn_36] -> Comparator35/2
  Comparator30/1 -> [result_38]
  [dataIn_24] -> Comparator34/1
  [dataIn_24] -> Comparator29/1
  [dataIn_37] -> Comparator29/2
  [dataIn_38] -> Comparator30/2
  Comparator33/1 -> [result_34]
  [result_13] -> Logical Bit Operator2/4
  [result_17] -> Logical Bit Operator2/8
  [result_14] -> Logical Bit Operator2/5
  [result_15] -> Logical Bit Operator2/6
  [result_16] -> Logical Bit Operator2/7
  [result_18] -> Logical Bit Operator2/9
  [result_12] -> Logical Bit Operator2/3
  Constant/1 -> Comparator6/1
  Logical Bit Operator/1 -> [result_24]
  Logical Bit Operator2/1 -> [isKeyPoint]
  Constant1/1 -> Comparator7/2
  Comparator6/1 -> Logical Bit Operator/1
  [dataIn_24] -> Comparator12/1
  [dataIn_25] -> Comparator19/2
  Comparator13/1 -> [result_21]
  Comparator19/1 -> [result_25]
  [dataIn_24] -> Comparator19/1
  [dataIn_20] -> Comparator12/2
  [dataIn_24] -> Comparator16/1
  [dataIn_24] -> Comparator14/1
  [dataIn_24] -> Comparator13/1
  Comparator16/1 -> [result_22]
  [dataIn_22] -> Comparator16/2
  Comparator14/1 -> [result_27]
  [dataIn_24] -> Comparator17/1
  [dataIn_23] -> Comparator17/2
  [dataIn_24] -> Comparator15/1
  [dataIn_27] -> Comparator14/2
  Comparator17/1 -> [result_23]
  [dataIn_28] -> Comparator15/2
  [dataIn_26] -> Comparator20/2
  Comparator12/1 -> [result_20]
  [dataIn_24] -> Comparator20/1
  Comparator15/1 -> [result_28]
  Comparator20/1 -> [result_26]
  [dataIn_21] -> Comparator13/2
  [isKeyPoint] -> is_KeyPoint/1
  dataIn_12/1 -> [dataIn_12]
  dataIn_13/1 -> [dataIn_13]
  Comparator/1 -> [result_10]
  [result_28] -> Logical Bit Operator2/18
  [result_30] -> Logical Bit Operator2/19
  [result_31] -> Logical Bit Operator2/20
  [result_33] -> Logical Bit Operator2/22
  [result_34] -> Logical Bit Operator2/23
  [result_36] -> Logical Bit Operator2/25
  [result_35] -> Logical Bit Operator2/24
  [result_32] -> Logical Bit Operator2/21
  [result_37] -> Logical Bit Operator2/26
  [result_38] -> Logical Bit Operator2/27
  [result_26] -> Logical Bit Operator2/16
  [result_25] -> Logical Bit Operator2/15
  [result_27] -> Logical Bit Operator2/17
  [result_24] -> Logical Bit Operator2/14
